simulink model "QuadcopterDynamicModel"  (R2023b)
settings: Solver=VariableStepAuto  StartTime=0.0  StopTime=10.0  RelTol=1e-3
settings Model: Creator=DELL  LastModifiedBy=DELL

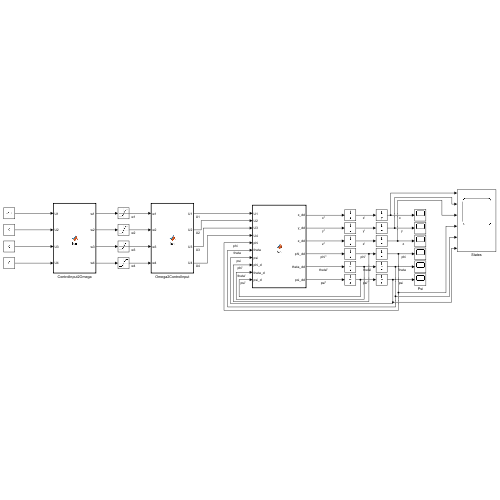
[thumbnail: Simulink's stored preview of the top-level diagram]
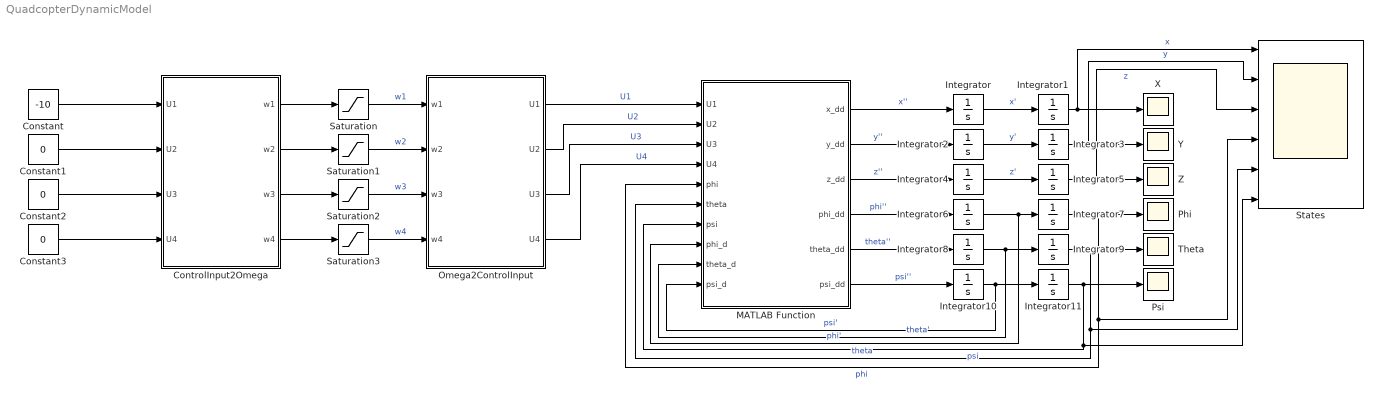
== system QuadcopterDynamicModel ==
  Constant : Constant  Value=-10
  Constant1 : Constant  Value=0
  Constant2 : Constant  Value=0
  Constant3 : Constant  Value=0
  ControlInput2Omega : MATLAB Function  TreatAsAtomicUnit=on
  Integrator{,1..11} (12 alike) : Integrator
  MATLAB Function : MATLAB Function  TreatAsAtomicUnit=on
  Omega2ControlInput : MATLAB Function  TreatAsAtomicUnit=on
  Phi : Scope
  Psi : Scope
  Saturation{,1..3} (4 alike) : Saturate  UpperLimit=550  LowerLimit=0
  States : Scope  NumInputPorts=6
  Theta : Scope
  X : Scope
  Y : Scope
  Z : Scope
  wires:
  ControlInput2Omega/2(w2) -> Saturation1/1
  ControlInput2Omega/1(w1) -> Saturation/1
  ControlInput2Omega/3(w3) -> Saturation2/1
  ControlInput2Omega/4(w4) -> Saturation3/1
  Integrator/1 -> Integrator1/1  "x'"
  Integrator2/1 -> Integrator3/1  "y'"
  Integrator4/1 -> Integrator5/1  "z'"
  Integrator6/1 -> MATLAB Function/8(phi_d), Integrator7/1  "phi'"
  Integrator8/1 -> MATLAB Function/9(theta_d), Integrator9/1  "theta'"
  Integrator10/1 -> MATLAB Function/10(psi_d), Integrator11/1  "psi'"
  Integrator1/1 -> States/1, X/1  "x"
  Integrator3/1 -> States/2, Y/1  "y"
  Integrator5/1 -> States/3, Z/1  "z"
  Integrator7/1 -> MATLAB Function/5(phi), States/4, Phi/1  "phi"
  Integrator9/1 -> Theta/1, MATLAB Function/6(theta), States/5  "theta"
  Integrator11/1 -> Psi/1, MATLAB Function/7(psi), States/6  "psi"
  Constant/1 -> ControlInput2Omega/1(U1)
  Constant1/1 -> ControlInput2Omega/2(U2)
  MATLAB Function/1(x_dd) -> Integrator/1  "x''"
  MATLAB Function/2(y_dd) -> Integrator2/1  "y''"
  MATLAB Function/3(z_dd) -> Integrator4/1  "z''"
  MATLAB Function/4(phi_dd) -> Integrator6/1  "phi''"
  MATLAB Function/5(theta_dd) -> Integrator8/1  "theta''"
  MATLAB Function/6(psi_dd) -> Integrator10/1  "psi''"
  Omega2ControlInput/1(U1) -> MATLAB Function/1(U1)  "U1"
  Omega2ControlInput/2(U2) -> MATLAB Function/2(U2)  "U2"
  Omega2ControlInput/3(U3) -> MATLAB Function/3(U3)  "U3"
  Omega2ControlInput/4(U4) -> MATLAB Function/4(U4)  "U4"
  Constant2/1 -> ControlInput2Omega/3(U3)
  Constant3/1 -> ControlInput2Omega/4(U4)
  Saturation/1 -> Omega2ControlInput/1(w1)  "w1"
  Saturation1/1 -> Omega2ControlInput/2(w2)  "w2"
  Saturation2/1 -> Omega2ControlInput/3(w3)  "w3"
  Saturation3/1 -> Omega2ControlInput/4(w4)  "w4"

== matlab function QuadcopterDynamicModel/Omega2ControlInput ==
  data: w1 input; U1 output; w2 input; w3 input; w4 input; U2 output; U3 output; U4 output
function [U1,U2,U3,U4] = fcn(w1,w2,w3,w4)
    
    % COEFFITIENTS
    Kf = 3.13e-5;
    Km = 7.5e-7;

    U1 = Kf * ((w1^2)+(w2^2)+(w3^2)+(w4^2));
    U2 = Kf * (-(w2^2)+(w4^2));
    U3 = Kf * ((w1^2)-(w3^2));
    U4 = Km * ((w1^2)-(w2^2)+(w3^2)-(w4^2));

== matlab function QuadcopterDynamicModel/MATLAB Function ==
  data: U1 input; x_dd output; U2 input; U3 input; U4 input; phi input; theta input; psi input; phi_d input; theta_d input; psi_d input; y_dd output; z_dd output; phi_dd output; theta_dd output; psi_dd output
function [x_dd,y_dd,z_dd,phi_dd,theta_dd,psi_dd] = fcn(U1,U2,U3,U4, phi,theta,psi, phi_d, theta_d, psi_d)
    
    % MOMENTS OF INERTIA
    Ixx = 7.5e-3;
    Iyy = 7.5e-3;
    Izz = 1.3e-2;
    
    % GYRO
    Jr = 0;
    wr = 0;
    
    % LENGTH
    l = 0.23;
    
    % MASS & GRAVITATIONAL ACCELERATION
    m = 0.65;
    g = 9.81;
    
    x_dd = -(U1/m)*(sin(phi)*sin(psi)+cos(phi)*cos(psi)*sin(theta));
    y_dd = -(U1/m)*(cos(phi)*sin(psi)*sin(theta)-cos(psi)*sin(phi));
    z_dd = g - (U1/m)*(cos(phi)*cos(theta));

    phi_dd = (l/Ixx)*U2 - (Jr/Ixx)*theta_d*wr + (Iyy/Ixx)*psi_d*theta_d - (Izz/Ixx)*theta_d*psi_d;
    theta_dd = (l/Iyy)*U3 - (Jr/Iyy)*phi_d*wr + (Izz/Iyy)*phi_d*psi_d - (Ixx/Iyy)*psi_d*phi_d;
    psi_dd = (1/Izz)*U4 + (Ixx/Izz)*theta_d*phi_d - (Iyy/Izz)*phi_d*theta_d;

y = [x_dd,y_dd,z_dd,phi_dd,theta_dd,psi_dd];

== matlab function QuadcopterDynamicModel/ControlInput2Omega ==
  data: U1 input; w1 output; U2 input; U3 input; U4 input; w2 output; w3 output; w4 output
function [w1,w2,w3,w4] = fcn(U1,U2,U3,U4)

    % COEFFITIENTS
    Kf = 3.13e-5;
    Km = 7.5e-7;

    w1 = abs((((U1/4)+(U3/2))/Kf + U4/(4*Km)))^(1/2);
    w2 = abs((((U1/4)-(U2/2))/Kf - U4/(4*Km)))^(1/2);
    w3 = abs((((U1/4)-(U3/2))/Kf + U4/(4*Km)))^(1/2);
    w4 = abs((((U1/4)+(U2/2))/Kf - U4/(4*Km)))^(1/2);

    % w1 = sqrt(abs((U1/(4*Kf))+(U3/(2*Kf))+(U4/(4*Km))));
    % w2 = sqrt(abs((U1/(4*Kf))-(U2/(2*Kf))-(U4/(4*Km))));
    % w3 = sqrt(abs((U1/(4*Kf))-(U3/(2*Kf))-(U4/(4*Km))));
    % w4 = sqrt(abs((U1/(4*Kf))+(U2/(2*Kf))-(U4/(4*Km))));
